simulink model "MATE_9LevelDrive_LowHarmonicRectifier"  (R2024b)
settings: Solver=FixedStepDiscrete  StartTime=0.0  StopTime=1  FixedStep=Ts  RelTol=1e-3
PostLoadFcn:
  | Ts=25e-6; initDrive9Level;Rsnu=30; Csnu=3e-6;Ron=0.01;Roff=1e6; Vf=2;
InitFcn:
  | Ts=25e-6; initDrive9Level;Rsnu=30; Csnu=3e-6;Ron=0.01;Roff=1e6; Vf=2;
values from neighbouring files (symbols this model uses):
  Lbase = Zbase/wbase    (= 0.0044902914611)    [initDrive9Level.m]
  Rgnd_rectifier = 1e4    (= 10000)    [initDrive9Level.m]
  T_2wind_ratio = 0.2677    [initDrive9Level.m]
  T_Lpu = Ltot_pu*9/10    (= 0.036)    [initDrive9Level.m]
  T_Lpu_pri = Ltot_pu/10    (= 0.004)    [initDrive9Level.m]
  T_Rpu = Rtot_pu*9/10    (= 0.009)    [initDrive9Level.m]
  T_Rpu_pri = Rtot_pu/10    (= 0.001)    [initDrive9Level.m]
  T_Vpri = 3000    [initDrive9Level.m]
  T_Vpri_15comp = 1.1168    [initDrive9Level.m]
  T_Vsec = 920    [initDrive9Level.m]
  Zbase = T_Vsec*T_Vsec/T_Pbase    (= 1.6928)    [initDrive9Level.m]
undefined symbols (not defined in the file or in its folder): DiscIntNeverNeededParam, gcbh, sps_rtmsupport
libraries: fl_lib x192, ee_lib x105, simetranss x26, nesl_utility x21
(part 3 of 5)

== system MATE_9LevelDrive_LowHarmonicRectifier/SSC multiwinding tranformer ==
  Electrical Reference : fl_lib/Electrical/Electrical Elements/Electrical Reference
  Electrical Reference1 : fl_lib/Electrical/Electrical Elements/Electrical Reference
  Electrical Reference2 : fl_lib/Electrical/Electrical Elements/Electrical Reference
  Phase Splitter{,4..7} (5 alike) : ee_lib/Connectors & References/Phase Splitter
  Seven-winding Decoupling Transformer : simetranss/Network decoupling/Seven-winding Decoupling Transformer  Tag=PublishSubsystem  Vpri=T_Vpri/sqrt(3)  RLpri=[T_Rpu_pri*Zbase T_Lpu_pri*Lbase]  Vwdn="[ T_Vsec/sqrt(3) T_Vsec T_Vsec/sqrt(3)*T_Vpri_15comp T_Vsec/sqrt(3)*T_2wind_ratio*T_Vpri_15comp T_Vsec/sqrt(3)*T_Vpri_15comp T_Vsec/sqrt(3)*T_2wind_ratio*T_Vpri_15comp  ]"  Lwdn="[T_Lpu_pri   T_Lpu T_Lpu T_Lpu*T_Vpri_15comp  T_Lpu*T_2wind_ratio*T_Vpri_15comp T_Lpu*T_Vpri_15comp  T_Lpu*T_2wind_ratio*T_Vpri_15comp ]*Lbase"  Rwdn="[     T_Rpu            T_Rpu    T_Rpu*T_Vpri_15comp T_Rpu*T_2wind_ratio*T_Vpri_15comp T_Rpu*T_Vpri_15comp T_Rpu*T_2wind_ratio*T_Vpri_15comp]*Zbase"  Rearth=1e6  Ts=Ts
  Seven-winding Decoupling Transformer1 : simetranss/Network decoupling/Seven-winding Decoupling Transformer  Tag=PublishSubsystem  Vpri=T_Vpri/sqrt(3)  RLpri=[T_Rpu_pri*Zbase T_Lpu_pri*Lbase]  Vwdn="[ T_Vsec/sqrt(3) T_Vsec T_Vsec/sqrt(3)*T_Vpri_15comp T_Vsec/sqrt(3)*T_2wind_ratio*T_Vpri_15comp T_Vsec/sqrt(3)*T_Vpri_15comp T_Vsec/sqrt(3)*T_2wind_ratio*T_Vpri_15comp  ]"  Lwdn="[T_Lpu_pri   T_Lpu T_Lpu T_Lpu*T_Vpri_15comp  T_Lpu*T_2wind_ratio*T_Vpri_15comp T_Lpu*T_Vpri_15comp  T_Lpu*T_2wind_ratio*T_Vpri_15comp ]*Lbase"  Rwdn="[     T_Rpu            T_Rpu    T_Rpu*T_Vpri_15comp T_Rpu*T_2wind_ratio*T_Vpri_15comp T_Rpu*T_Vpri_15comp T_Rpu*T_2wind_ratio*T_Vpri_15comp]*Zbase"  Rearth=1e6  Ts=Ts
  Seven-winding Decoupling Transformer2 : simetranss/Network decoupling/Seven-winding Decoupling Transformer  Tag=PublishSubsystem  Vpri=T_Vpri/sqrt(3)  RLpri=[T_Rpu_pri*Zbase T_Lpu_pri*Lbase]  Vwdn="[ T_Vsec/sqrt(3) T_Vsec T_Vsec/sqrt(3)*T_Vpri_15comp T_Vsec/sqrt(3)*T_2wind_ratio*T_Vpri_15comp T_Vsec/sqrt(3)*T_Vpri_15comp T_Vsec/sqrt(3)*T_2wind_ratio*T_Vpri_15comp  ]"  Lwdn="[T_Lpu_pri   T_Lpu T_Lpu T_Lpu*T_Vpri_15comp  T_Lpu*T_2wind_ratio*T_Vpri_15comp T_Lpu*T_Vpri_15comp  T_Lpu*T_2wind_ratio*T_Vpri_15comp ]*Lbase"  Rwdn="[     T_Rpu            T_Rpu    T_Rpu*T_Vpri_15comp T_Rpu*T_2wind_ratio*T_Vpri_15comp T_Rpu*T_Vpri_15comp T_Rpu*T_2wind_ratio*T_Vpri_15comp]*Zbase"  Rearth=1e6  Ts=Ts
  abc : PMIOPort  Side=Left
  abc2 : PMIOPort  Port=2  Side=Right
  abc3 : PMIOPort  Port=3  Side=Right
  abc4 : PMIOPort  Port=4  Side=Right
  abc5 : PMIOPort  Port=5  Side=Right
  connections:
  Seven-winding Decoupling Transformer/LConn2 -- Electrical Reference/LConn1
  Seven-winding Decoupling Transformer1/LConn2 -- Electrical Reference1/LConn1
  Seven-winding Decoupling Transformer2/LConn2 -- Electrical Reference2/LConn1
  Seven-winding Decoupling Transformer1/RConn8 -- Seven-winding Decoupling Transformer/RConn8 -- Seven-winding Decoupling Transformer2/RConn8
  Phase Splitter6/RConn2 -- Seven-winding Decoupling Transformer1/RConn5
  Phase Splitter6/RConn3 -- Seven-winding Decoupling Transformer2/RConn5
  Phase Splitter5/RConn2 -- Seven-winding Decoupling Transformer1/RConn1
  Phase Splitter5/RConn3 -- Seven-winding Decoupling Transformer2/RConn1
  Phase Splitter5/RConn1 -- Seven-winding Decoupling Transformer/RConn1
  Seven-winding Decoupling Transformer1/RConn2 -- Seven-winding Decoupling Transformer/RConn2 -- Seven-winding Decoupling Transformer2/RConn2
  Seven-winding Decoupling Transformer2/RConn6 -- Seven-winding Decoupling Transformer/RConn7
  Seven-winding Decoupling Transformer2/RConn3 -- Seven-winding Decoupling Transformer1/RConn4 -- Phase Splitter4/RConn3
  Seven-winding Decoupling Transformer1/RConn12 -- Seven-winding Decoupling Transformer/RConn12 -- Seven-winding Decoupling Transformer2/RConn12
  Phase Splitter7/RConn1 -- Seven-winding Decoupling Transformer/RConn9
  Phase Splitter7/RConn2 -- Seven-winding Decoupling Transformer1/RConn9
  Phase Splitter7/RConn3 -- Seven-winding Decoupling Transformer2/RConn9
  Seven-winding Decoupling Transformer2/RConn10 -- Seven-winding Decoupling Transformer1/RConn11
  Seven-winding Decoupling Transformer1/RConn10 -- Seven-winding Decoupling Transformer/RConn11
  Seven-winding Decoupling Transformer2/RConn11 -- Seven-winding Decoupling Transformer/RConn10
  Seven-winding Decoupling Transformer1/RConn3 -- Seven-winding Decoupling Transformer/RConn4 -- Phase Splitter4/RConn2
  Seven-winding Decoupling Transformer2/RConn4 -- Seven-winding Decoupling Transformer/RConn3 -- Phase Splitter4/RConn1
  Seven-winding Decoupling Transformer1/RConn7 -- Seven-winding Decoupling Transformer/RConn6
  Phase Splitter6/RConn1 -- Seven-winding Decoupling Transformer/RConn5
  Seven-winding Decoupling Transformer2/RConn7 -- Seven-winding Decoupling Transformer1/RConn6
  Phase Splitter/RConn1 -- Seven-winding Decoupling Transformer/LConn1
  Seven-winding Decoupling Transformer1/LConn1 -- Phase Splitter/RConn2
  Phase Splitter/RConn3 -- Seven-winding Decoupling Transformer2/LConn1
  abc2/RConn1 -- Phase Splitter5/LConn1
  abc3/RConn1 -- Phase Splitter4/LConn1
  abc4/RConn1 -- Phase Splitter6/LConn1
  abc5/RConn1 -- Phase Splitter7/LConn1
  abc/RConn1 -- Phase Splitter/LConn1

== system MATE_9LevelDrive_LowHarmonicRectifier/SSC multiwinding tranformer1 ==
  Electrical Reference : fl_lib/Electrical/Electrical Elements/Electrical Reference
  Electrical Reference1 : fl_lib/Electrical/Electrical Elements/Electrical Reference
  Electrical Reference2 : fl_lib/Electrical/Electrical Elements/Electrical Reference
  Phase Splitter{,4..7} (5 alike) : ee_lib/Connectors & References/Phase Splitter
  Seven-winding Decoupling Transformer : simetranss/Network decoupling/Seven-winding Decoupling Transformer  Tag=PublishSubsystem  Vpri=T_Vpri/sqrt(3)  RLpri=[T_Rpu_pri*Zbase T_Lpu_pri*Lbase]  Vwdn="[ T_Vsec/sqrt(3) T_Vsec T_Vsec/sqrt(3)*T_Vpri_15comp T_Vsec/sqrt(3)*T_2wind_ratio*T_Vpri_15comp T_Vsec/sqrt(3)*T_Vpri_15comp T_Vsec/sqrt(3)*T_2wind_ratio*T_Vpri_15comp  ]"  Lwdn="[T_Lpu_pri   T_Lpu T_Lpu T_Lpu*T_Vpri_15comp  T_Lpu*T_2wind_ratio*T_Vpri_15comp T_Lpu*T_Vpri_15comp  T_Lpu*T_2wind_ratio*T_Vpri_15comp ]*Lbase"  Rwdn="[     T_Rpu            T_Rpu    T_Rpu*T_Vpri_15comp T_Rpu*T_2wind_ratio*T_Vpri_15comp T_Rpu*T_Vpri_15comp T_Rpu*T_2wind_ratio*T_Vpri_15comp]*Zbase"  Rearth=1e6  Ts=Ts
  Seven-winding Decoupling Transformer1 : simetranss/Network decoupling/Seven-winding Decoupling Transformer  Tag=PublishSubsystem  Vpri=T_Vpri/sqrt(3)  RLpri=[T_Rpu_pri*Zbase T_Lpu_pri*Lbase]  Vwdn="[ T_Vsec/sqrt(3) T_Vsec T_Vsec/sqrt(3)*T_Vpri_15comp T_Vsec/sqrt(3)*T_2wind_ratio*T_Vpri_15comp T_Vsec/sqrt(3)*T_Vpri_15comp T_Vsec/sqrt(3)*T_2wind_ratio*T_Vpri_15comp  ]"  Lwdn="[T_Lpu_pri   T_Lpu T_Lpu T_Lpu*T_Vpri_15comp  T_Lpu*T_2wind_ratio*T_Vpri_15comp T_Lpu*T_Vpri_15comp  T_Lpu*T_2wind_ratio*T_Vpri_15comp ]*Lbase"  Rwdn="[     T_Rpu            T_Rpu    T_Rpu*T_Vpri_15comp T_Rpu*T_2wind_ratio*T_Vpri_15comp T_Rpu*T_Vpri_15comp T_Rpu*T_2wind_ratio*T_Vpri_15comp]*Zbase"  Rearth=1e6  Ts=Ts
  Seven-winding Decoupling Transformer2 : simetranss/Network decoupling/Seven-winding Decoupling Transformer  Tag=PublishSubsystem  Vpri=T_Vpri/sqrt(3)  RLpri=[T_Rpu_pri*Zbase T_Lpu_pri*Lbase]  Vwdn="[ T_Vsec/sqrt(3) T_Vsec T_Vsec/sqrt(3)*T_Vpri_15comp T_Vsec/sqrt(3)*T_2wind_ratio*T_Vpri_15comp T_Vsec/sqrt(3)*T_Vpri_15comp T_Vsec/sqrt(3)*T_2wind_ratio*T_Vpri_15comp  ]"  Lwdn="[T_Lpu_pri   T_Lpu T_Lpu T_Lpu*T_Vpri_15comp  T_Lpu*T_2wind_ratio*T_Vpri_15comp T_Lpu*T_Vpri_15comp  T_Lpu*T_2wind_ratio*T_Vpri_15comp ]*Lbase"  Rwdn="[     T_Rpu            T_Rpu    T_Rpu*T_Vpri_15comp T_Rpu*T_2wind_ratio*T_Vpri_15comp T_Rpu*T_Vpri_15comp T_Rpu*T_2wind_ratio*T_Vpri_15comp]*Zbase"  Rearth=1e6  Ts=Ts
  abc : PMIOPort  Side=Left
  abc2 : PMIOPort  Port=2  Side=Right
  abc3 : PMIOPort  Port=3  Side=Right
  abc4 : PMIOPort  Port=4  Side=Right
  abc5 : PMIOPort  Port=5  Side=Right
  connections:
  abc5/RConn1 -- Phase Splitter7/LConn1
  abc4/RConn1 -- Phase Splitter6/LConn1
  abc3/RConn1 -- Phase Splitter4/LConn1
  abc2/RConn1 -- Phase Splitter5/LConn1
  Phase Splitter/RConn3 -- Seven-winding Decoupling Transformer2/LConn1
  Seven-winding Decoupling Transformer1/LConn1 -- Phase Splitter/RConn2
  Phase Splitter/RConn1 -- Seven-winding Decoupling Transformer/LConn1
  Seven-winding Decoupling Transformer2/RConn7 -- Seven-winding Decoupling Transformer1/RConn6
  Phase Splitter6/RConn1 -- Seven-winding Decoupling Transformer/RConn5
  Seven-winding Decoupling Transformer1/RConn7 -- Seven-winding Decoupling Transformer/RConn6
  Phase Splitter4/RConn1 -- Seven-winding Decoupling Transformer/RConn3 -- Seven-winding Decoupling Transformer2/RConn4
  Phase Splitter4/RConn2 -- Seven-winding Decoupling Transformer/RConn4 -- Seven-winding Decoupling Transformer1/RConn3
  Seven-winding Decoupling Transformer2/RConn11 -- Seven-winding Decoupling Transformer/RConn10
  Seven-winding Decoupling Transformer1/RConn10 -- Seven-winding Decoupling Transformer/RConn11
  Seven-winding Decoupling Transformer2/RConn10 -- Seven-winding Decoupling Transformer1/RConn11
  Phase Splitter7/RConn3 -- Seven-winding Decoupling Transformer2/RConn9
  Phase Splitter7/RConn2 -- Seven-winding Decoupling Transformer1/RConn9
  Phase Splitter7/RConn1 -- Seven-winding Decoupling Transformer/RConn9
  Seven-winding Decoupling Transformer2/RConn12 -- Seven-winding Decoupling Transformer/RConn12 -- Seven-winding Decoupling Transformer1/RConn12
  Phase Splitter4/RConn3 -- Seven-winding Decoupling Transformer1/RConn4 -- Seven-winding Decoupling Transformer2/RConn3
  Seven-winding Decoupling Transformer2/RConn6 -- Seven-winding Decoupling Transformer/RConn7
  Seven-winding Decoupling Transformer2/RConn2 -- Seven-winding Decoupling Transformer/RConn2 -- Seven-winding Decoupling Transformer1/RConn2
  Phase Splitter5/RConn1 -- Seven-winding Decoupling Transformer/RConn1
  Phase Splitter5/RConn3 -- Seven-winding Decoupling Transformer2/RConn1
  Phase Splitter5/RConn2 -- Seven-winding Decoupling Transformer1/RConn1
  Phase Splitter6/RConn3 -- Seven-winding Decoupling Transformer2/RConn5
  Phase Splitter6/RConn2 -- Seven-winding Decoupling Transformer1/RConn5
  Seven-winding Decoupling Transformer2/RConn8 -- Seven-winding Decoupling Transformer/RConn8 -- Seven-winding Decoupling Transformer1/RConn8
  Seven-winding Decoupling Transformer2/LConn2 -- Electrical Reference2/LConn1
  Seven-winding Decoupling Transformer1/LConn2 -- Electrical Reference1/LConn1
  Seven-winding Decoupling Transformer/LConn2 -- Electrical Reference/LConn1
  abc/RConn1 -- Phase Splitter/LConn1

== system MATE_9LevelDrive_LowHarmonicRectifier/SSC multiwinding tranformer2 ==
  Electrical Reference : fl_lib/Electrical/Electrical Elements/Electrical Reference
  Electrical Reference1 : fl_lib/Electrical/Electrical Elements/Electrical Reference
  Electrical Reference2 : fl_lib/Electrical/Electrical Elements/Electrical Reference
  Phase Splitter{,4..7} (5 alike) : ee_lib/Connectors & References/Phase Splitter
  Seven-winding Decoupling Transformer : simetranss/Network decoupling/Seven-winding Decoupling Transformer  Tag=PublishSubsystem  Vpri=T_Vpri/sqrt(3)  RLpri=[T_Rpu_pri*Zbase T_Lpu_pri*Lbase]  Vwdn="[ T_Vsec/sqrt(3) T_Vsec T_Vsec/sqrt(3)*T_Vpri_15comp T_Vsec/sqrt(3)*T_2wind_ratio*T_Vpri_15comp T_Vsec/sqrt(3)*T_Vpri_15comp T_Vsec/sqrt(3)*T_2wind_ratio*T_Vpri_15comp  ]"  Lwdn="[T_Lpu_pri   T_Lpu T_Lpu T_Lpu*T_Vpri_15comp  T_Lpu*T_2wind_ratio*T_Vpri_15comp T_Lpu*T_Vpri_15comp  T_Lpu*T_2wind_ratio*T_Vpri_15comp ]*Lbase"  Rwdn="[     T_Rpu            T_Rpu    T_Rpu*T_Vpri_15comp T_Rpu*T_2wind_ratio*T_Vpri_15comp T_Rpu*T_Vpri_15comp T_Rpu*T_2wind_ratio*T_Vpri_15comp]*Zbase"  Rearth=1e6  Ts=Ts
  Seven-winding Decoupling Transformer1 : simetranss/Network decoupling/Seven-winding Decoupling Transformer  Tag=PublishSubsystem  Vpri=T_Vpri/sqrt(3)  RLpri=[T_Rpu_pri*Zbase T_Lpu_pri*Lbase]  Vwdn="[ T_Vsec/sqrt(3) T_Vsec T_Vsec/sqrt(3)*T_Vpri_15comp T_Vsec/sqrt(3)*T_2wind_ratio*T_Vpri_15comp T_Vsec/sqrt(3)*T_Vpri_15comp T_Vsec/sqrt(3)*T_2wind_ratio*T_Vpri_15comp  ]"  Lwdn="[T_Lpu_pri   T_Lpu T_Lpu T_Lpu*T_Vpri_15comp  T_Lpu*T_2wind_ratio*T_Vpri_15comp T_Lpu*T_Vpri_15comp  T_Lpu*T_2wind_ratio*T_Vpri_15comp ]*Lbase"  Rwdn="[     T_Rpu            T_Rpu    T_Rpu*T_Vpri_15comp T_Rpu*T_2wind_ratio*T_Vpri_15comp T_Rpu*T_Vpri_15comp T_Rpu*T_2wind_ratio*T_Vpri_15comp]*Zbase"  Rearth=1e6  Ts=Ts
  Seven-winding Decoupling Transformer2 : simetranss/Network decoupling/Seven-winding Decoupling Transformer  Tag=PublishSubsystem  Vpri=T_Vpri/sqrt(3)  RLpri=[T_Rpu_pri*Zbase T_Lpu_pri*Lbase]  Vwdn="[ T_Vsec/sqrt(3) T_Vsec T_Vsec/sqrt(3)*T_Vpri_15comp T_Vsec/sqrt(3)*T_2wind_ratio*T_Vpri_15comp T_Vsec/sqrt(3)*T_Vpri_15comp T_Vsec/sqrt(3)*T_2wind_ratio*T_Vpri_15comp  ]"  Lwdn="[T_Lpu_pri   T_Lpu T_Lpu T_Lpu*T_Vpri_15comp  T_Lpu*T_2wind_ratio*T_Vpri_15comp T_Lpu*T_Vpri_15comp  T_Lpu*T_2wind_ratio*T_Vpri_15comp ]*Lbase"  Rwdn="[     T_Rpu            T_Rpu    T_Rpu*T_Vpri_15comp T_Rpu*T_2wind_ratio*T_Vpri_15comp T_Rpu*T_Vpri_15comp T_Rpu*T_2wind_ratio*T_Vpri_15comp]*Zbase"  Rearth=1e6  Ts=Ts
  abc : PMIOPort  Side=Left
  abc2 : PMIOPort  Port=2  Side=Right
  abc3 : PMIOPort  Port=3  Side=Right
  abc4 : PMIOPort  Port=4  Side=Right
  abc5 : PMIOPort  Port=5  Side=Right
  connections:
  Seven-winding Decoupling Transformer/LConn2 -- Electrical Reference/LConn1
  Seven-winding Decoupling Transformer1/LConn2 -- Electrical Reference1/LConn1
  Seven-winding Decoupling Transformer2/LConn2 -- Electrical Reference2/LConn1
  Seven-winding Decoupling Transformer1/RConn8 -- Seven-winding Decoupling Transformer/RConn8 -- Seven-winding Decoupling Transformer2/RConn8
  Phase Splitter6/RConn2 -- Seven-winding Decoupling Transformer1/RConn5
  Phase Splitter6/RConn3 -- Seven-winding Decoupling Transformer2/RConn5
  Phase Splitter5/RConn2 -- Seven-winding Decoupling Transformer1/RConn1
  Phase Splitter5/RConn3 -- Seven-winding Decoupling Transformer2/RConn1
  Phase Splitter5/RConn1 -- Seven-winding Decoupling Transformer/RConn1
  Seven-winding Decoupling Transformer1/RConn2 -- Seven-winding Decoupling Transformer/RConn2 -- Seven-winding Decoupling Transformer2/RConn2
  Seven-winding Decoupling Transformer2/RConn6 -- Seven-winding Decoupling Transformer/RConn7
  Seven-winding Decoupling Transformer2/RConn3 -- Seven-winding Decoupling Transformer1/RConn4 -- Phase Splitter4/RConn3
  Seven-winding Decoupling Transformer1/RConn12 -- Seven-winding Decoupling Transformer/RConn12 -- Seven-winding Decoupling Transformer2/RConn12
  Phase Splitter7/RConn1 -- Seven-winding Decoupling Transformer/RConn9
  Phase Splitter7/RConn2 -- Seven-winding Decoupling Transformer1/RConn9
  Phase Splitter7/RConn3 -- Seven-winding Decoupling Transformer2/RConn9
  Seven-winding Decoupling Transformer2/RConn10 -- Seven-winding Decoupling Transformer1/RConn11
  Seven-winding Decoupling Transformer1/RConn10 -- Seven-winding Decoupling Transformer/RConn11
  Seven-winding Decoupling Transformer2/RConn11 -- Seven-winding Decoupling Transformer/RConn10
  Seven-winding Decoupling Transformer1/RConn3 -- Seven-winding Decoupling Transformer/RConn4 -- Phase Splitter4/RConn2
  Seven-winding Decoupling Transformer2/RConn4 -- Seven-winding Decoupling Transformer/RConn3 -- Phase Splitter4/RConn1
  Seven-winding Decoupling Transformer1/RConn7 -- Seven-winding Decoupling Transformer/RConn6
  Phase Splitter6/RConn1 -- Seven-winding Decoupling Transformer/RConn5
  Seven-winding Decoupling Transformer2/RConn7 -- Seven-winding Decoupling Transformer1/RConn6
  Phase Splitter/RConn1 -- Seven-winding Decoupling Transformer/LConn1
  Seven-winding Decoupling Transformer1/LConn1 -- Phase Splitter/RConn2
  Phase Splitter/RConn3 -- Seven-winding Decoupling Transformer2/LConn1
  abc2/RConn1 -- Phase Splitter5/LConn1
  abc3/RConn1 -- Phase Splitter4/LConn1
  abc4/RConn1 -- Phase Splitter6/LConn1
  abc5/RConn1 -- Phase Splitter7/LConn1
  abc/RConn1 -- Phase Splitter/LConn1

== system MATE_9LevelDrive_LowHarmonicRectifier/Subsystem1 ==
  Electrical Reference1 : fl_lib/Electrical/Electrical Elements/Electrical Reference
  Resistor : fl_lib/Electrical/Electrical Elements/Resistor  R=Rr Ohm  i_specify=off  i_priority=None  i=0 A  i_nominal_specify=off  i_nominal_value=1  i_nominal_unit=A  v_specify=off  v_priority=None  v=0 V  v_nominal_specify=off  v_nominal_value=1  v_nominal_unit=V
  Conn1 : PMIOPort  Side=Right
  connections:
  Resistor/RConn1 -- Conn1/RConn1
  Electrical Reference1/LConn1 -- Resistor/LConn1

== system MATE_9LevelDrive_LowHarmonicRectifier/Subsystem10 ==
  Electrical Reference1 : fl_lib/Electrical/Electrical Elements/Electrical Reference
  Resistor : fl_lib/Electrical/Electrical Elements/Resistor  R=Rr Ohm  i_specify=off  i_priority=None  i=0 A  i_nominal_specify=off  i_nominal_value=1  i_nominal_unit=A  v_specify=off  v_priority=None  v=0 V  v_nominal_specify=off  v_nominal_value=1  v_nominal_unit=V
  Conn1 : PMIOPort  Side=Right
  connections:
  Resistor/RConn1 -- Conn1/RConn1
  Electrical Reference1/LConn1 -- Resistor/LConn1

== system MATE_9LevelDrive_LowHarmonicRectifier/Subsystem11 ==
  Electrical Reference1 : fl_lib/Electrical/Electrical Elements/Electrical Reference
  Resistor : fl_lib/Electrical/Electrical Elements/Resistor  R=Rr Ohm  i_specify=off  i_priority=None  i=0 A  i_nominal_specify=off  i_nominal_value=1  i_nominal_unit=A  v_specify=off  v_priority=None  v=0 V  v_nominal_specify=off  v_nominal_value=1  v_nominal_unit=V
  Conn1 : PMIOPort  Side=Right
  connections:
  Electrical Reference1/LConn1 -- Resistor/LConn1
  Resistor/RConn1 -- Conn1/RConn1

== system MATE_9LevelDrive_LowHarmonicRectifier/Subsystem12 ==
  Electrical Reference1 : fl_lib/Electrical/Electrical Elements/Electrical Reference
  Resistor : fl_lib/Electrical/Electrical Elements/Resistor  R=Rr Ohm  i_specify=off  i_priority=None  i=0 A  i_nominal_specify=off  i_nominal_value=1  i_nominal_unit=A  v_specify=off  v_priority=None  v=0 V  v_nominal_specify=off  v_nominal_value=1  v_nominal_unit=V
  Conn1 : PMIOPort  Side=Right
  connections:
  Resistor/RConn1 -- Conn1/RConn1
  Electrical Reference1/LConn1 -- Resistor/LConn1

== system MATE_9LevelDrive_LowHarmonicRectifier/Subsystem13 ==
  Electrical Reference1 : fl_lib/Electrical/Electrical Elements/Electrical Reference
  Resistor : fl_lib/Electrical/Electrical Elements/Resistor  R=Rr Ohm  i_specify=off  i_priority=None  i=0 A  i_nominal_specify=off  i_nominal_value=1  i_nominal_unit=A  v_specify=off  v_priority=None  v=0 V  v_nominal_specify=off  v_nominal_value=1  v_nominal_unit=V
  Conn1 : PMIOPort  Side=Right
  connections:
  Electrical Reference1/LConn1 -- Resistor/LConn1
  Resistor/RConn1 -- Conn1/RConn1

== system MATE_9LevelDrive_LowHarmonicRectifier/Subsystem14 ==
  Electrical Reference1 : fl_lib/Electrical/Electrical Elements/Electrical Reference
  Resistor : fl_lib/Electrical/Electrical Elements/Resistor  R=Rr Ohm  i_specify=off  i_priority=None  i=0 A  i_nominal_specify=off  i_nominal_value=1  i_nominal_unit=A  v_specify=off  v_priority=None  v=0 V  v_nominal_specify=off  v_nominal_value=1  v_nominal_unit=V
  Conn1 : PMIOPort  Side=Right
  connections:
  Resistor/RConn1 -- Conn1/RConn1
  Electrical Reference1/LConn1 -- Resistor/LConn1

== system MATE_9LevelDrive_LowHarmonicRectifier/Subsystem2 ==
  Electrical Reference1 : fl_lib/Electrical/Electrical Elements/Electrical Reference
  Resistor : fl_lib/Electrical/Electrical Elements/Resistor  R=Rr Ohm  i_specify=off  i_priority=None  i=0 A  i_nominal_specify=off  i_nominal_value=1  i_nominal_unit=A  v_specify=off  v_priority=None  v=0 V  v_nominal_specify=off  v_nominal_value=1  v_nominal_unit=V
  Conn1 : PMIOPort  Side=Right
  connections:
  Electrical Reference1/LConn1 -- Resistor/LConn1
  Resistor/RConn1 -- Conn1/RConn1

== system MATE_9LevelDrive_LowHarmonicRectifier/Subsystem3 ==
  Electrical Reference1 : fl_lib/Electrical/Electrical Elements/Electrical Reference
  Resistor : fl_lib/Electrical/Electrical Elements/Resistor  R=Rr Ohm  i_specify=off  i_priority=None  i=0 A  i_nominal_specify=off  i_nominal_value=1  i_nominal_unit=A  v_specify=off  v_priority=None  v=0 V  v_nominal_specify=off  v_nominal_value=1  v_nominal_unit=V
  Conn1 : PMIOPort  Side=Right
  connections:
  Electrical Reference1/LConn1 -- Resistor/LConn1
  Resistor/RConn1 -- Conn1/RConn1

== system MATE_9LevelDrive_LowHarmonicRectifier/Subsystem4 ==
  Electrical Reference1 : fl_lib/Electrical/Electrical Elements/Electrical Reference
  Resistor : fl_lib/Electrical/Electrical Elements/Resistor  R=Rr Ohm  i_specify=off  i_priority=None  i=0 A  i_nominal_specify=off  i_nominal_value=1  i_nominal_unit=A  v_specify=off  v_priority=None  v=0 V  v_nominal_specify=off  v_nominal_value=1  v_nominal_unit=V
  Conn1 : PMIOPort  Side=Right
  connections:
  Resistor/RConn1 -- Conn1/RConn1
  Electrical Reference1/LConn1 -- Resistor/LConn1

== system MATE_9LevelDrive_LowHarmonicRectifier/Subsystem6 ==
  Electrical Reference1 : fl_lib/Electrical/Electrical Elements/Electrical Reference
  Resistor : fl_lib/Electrical/Electrical Elements/Resistor  R=Rr Ohm  i_specify=off  i_priority=None  i=0 A  i_nominal_specify=off  i_nominal_value=1  i_nominal_unit=A  v_specify=off  v_priority=None  v=0 V  v_nominal_specify=off  v_nominal_value=1  v_nominal_unit=V
  Conn1 : PMIOPort  Side=Right
  connections:
  Resistor/RConn1 -- Conn1/RConn1
  Electrical Reference1/LConn1 -- Resistor/LConn1

== system MATE_9LevelDrive_LowHarmonicRectifier/Subsystem7 ==
  Electrical Reference1 : fl_lib/Electrical/Electrical Elements/Electrical Reference
  Resistor : fl_lib/Electrical/Electrical Elements/Resistor  R=Rr Ohm  i_specify=off  i_priority=None  i=0 A  i_nominal_specify=off  i_nominal_value=1  i_nominal_unit=A  v_specify=off  v_priority=None  v=0 V  v_nominal_specify=off  v_nominal_value=1  v_nominal_unit=V
  Conn1 : PMIOPort  Side=Right
  connections:
  Electrical Reference1/LConn1 -- Resistor/LConn1
  Resistor/RConn1 -- Conn1/RConn1

== system MATE_9LevelDrive_LowHarmonicRectifier/Subsystem8 ==
  Electrical Reference1 : fl_lib/Electrical/Electrical Elements/Electrical Reference
  Resistor : fl_lib/Electrical/Electrical Elements/Resistor  R=Rr Ohm  i_specify=off  i_priority=None  i=0 A  i_nominal_specify=off  i_nominal_value=1  i_nominal_unit=A  v_specify=off  v_priority=None  v=0 V  v_nominal_specify=off  v_nominal_value=1  v_nominal_unit=V
  Conn1 : PMIOPort  Side=Right
  connections:
  Resistor/RConn1 -- Conn1/RConn1
  Electrical Reference1/LConn1 -- Resistor/LConn1

== system MATE_9LevelDrive_LowHarmonicRectifier/Subsystem9 ==
  Electrical Reference1 : fl_lib/Electrical/Electrical Elements/Electrical Reference
  Resistor : fl_lib/Electrical/Electrical Elements/Resistor  R=Rr Ohm  i_specify=off  i_priority=None  i=0 A  i_nominal_specify=off  i_nominal_value=1  i_nominal_unit=A  v_specify=off  v_priority=None  v=0 V  v_nominal_specify=off  v_nominal_value=1  v_nominal_unit=V
  Conn1 : PMIOPort  Side=Right
  connections:
  Electrical Reference1/LConn1 -- Resistor/LConn1
  Resistor/RConn1 -- Conn1/RConn1

== system MATE_9LevelDrive_LowHarmonicRectifier/backEMF ==
  amp : Inport
  freq : Inport  Port=2
  Constant1 : Constant  Value=2*pi/3
  Discrete-Time Integrator : DiscreteIntegrator  SampleTime=Ts  ICPrevOutput=DiscIntNeverNeededParam  ICPrevScaledInput=DiscIntNeverNeededParam
  Gain3 : Gain  Gain=2*pi
  Mux6 : Mux  Inputs=3
  Product2 : Product  RndMeth=Zero
  Sum : Sum  Inputs=+-
  Sum1 : Sum
  Trigonometric Function : Trigonometry
  Trigonometric Function1 : Trigonometry
  Trigonometric Function2 : Trigonometry
  Out1 : Outport  VectorParamsAs1DForOutWhenUnconnected=off
  wires:
  amp/1 -> Product2/1
  Mux6/1 -> Product2/2
  Trigonometric Function/1 -> Mux6/1
  Sum1/1 -> Trigonometric Function2/1
  Constant1/1 -> Sum1/2, Sum/2
  Sum/1 -> Trigonometric Function1/1
  Gain3/1 -> Discrete-Time Integrator/1
  Discrete-Time Integrator/1 -> Sum1/1, Sum/1, Trigonometric Function/1
  Product2/1 -> Out1/1
  freq/1 -> Gain3/1
  Trigonometric Function2/1 -> Mux6/3
  Trigonometric Function1/1 -> Mux6/2

== system MATE_9LevelDrive_LowHarmonicRectifier/Diode Bridge with snubber1/RCsnuber ==
  Capacitor : fl_lib/Electrical/Electrical Elements/Capacitor  c=Csnu F  r=0 Ohm  g=0 1/Ohm  i_specify=off  i_priority=None  i=0 A  i_nominal_specify=off  i_nominal_value=1  i_nominal_unit=A  v_specify=off  v_priority=None  v=0 V  v_nominal_specify=off  v_nominal_value=1  v_nominal_unit=V  vc_specify=off  vc_priority=High  vc=0 V  vc_nominal_specify=off  vc_nominal_value=1  vc_nominal_unit=V
  Resistor : fl_lib/Electrical/Electrical Elements/Resistor  R=Rsnu Ohm  i_specify=off  i_priority=None  i=0 A  i_nominal_specify=off  i_nominal_value=1  i_nominal_unit=A  v_specify=off  v_priority=None  v=0 V  v_nominal_specify=off  v_nominal_value=1  v_nominal_unit=V
  + : PMIOPort  Side=Left
  - : PMIOPort  Port=2  Side=Right
  connections:
  Resistor/LConn1 -- Capacitor/RConn1
  Capacitor/LConn1 -- +/RConn1
  Resistor/RConn1 -- -/RConn1

== system MATE_9LevelDrive_LowHarmonicRectifier/Diode Bridge with snubber1/RCsnuber1 ==
  Capacitor : fl_lib/Electrical/Electrical Elements/Capacitor  c=Csnu F  r=0 Ohm  g=0 1/Ohm  i_specify=off  i_priority=None  i=0 A  i_nominal_specify=off  i_nominal_value=1  i_nominal_unit=A  v_specify=off  v_priority=None  v=0 V  v_nominal_specify=off  v_nominal_value=1  v_nominal_unit=V  vc_specify=off  vc_priority=High  vc=0 V  vc_nominal_specify=off  vc_nominal_value=1  vc_nominal_unit=V
  Resistor : fl_lib/Electrical/Electrical Elements/Resistor  R=Rsnu Ohm  i_specify=off  i_priority=None  i=0 A  i_nominal_specify=off  i_nominal_value=1  i_nominal_unit=A  v_specify=off  v_priority=None  v=0 V  v_nominal_specify=off  v_nominal_value=1  v_nominal_unit=V
  + : PMIOPort  Side=Left
  - : PMIOPort  Port=2  Side=Right
  connections:
  Resistor/RConn1 -- -/RConn1
  Capacitor/LConn1 -- +/RConn1
  Resistor/LConn1 -- Capacitor/RConn1

== system MATE_9LevelDrive_LowHarmonicRectifier/Diode Bridge with snubber1/RCsnuber2 ==
  Capacitor : fl_lib/Electrical/Electrical Elements/Capacitor  c=Csnu F  r=0 Ohm  g=0 1/Ohm  i_specify=off  i_priority=None  i=0 A  i_nominal_specify=off  i_nominal_value=1  i_nominal_unit=A  v_specify=off  v_priority=None  v=0 V  v_nominal_specify=off  v_nominal_value=1  v_nominal_unit=V  vc_specify=off  vc_priority=High  vc=0 V  vc_nominal_specify=off  vc_nominal_value=1  vc_nominal_unit=V
  Resistor : fl_lib/Electrical/Electrical Elements/Resistor  R=Rsnu Ohm  i_specify=off  i_priority=None  i=0 A  i_nominal_specify=off  i_nominal_value=1  i_nominal_unit=A  v_specify=off  v_priority=None  v=0 V  v_nominal_specify=off  v_nominal_value=1  v_nominal_unit=V
  + : PMIOPort  Side=Left
  - : PMIOPort  Port=2  Side=Right
  connections:
  Resistor/LConn1 -- Capacitor/RConn1
  Capacitor/LConn1 -- +/RConn1
  Resistor/RConn1 -- -/RConn1

== system MATE_9LevelDrive_LowHarmonicRectifier/Diode Bridge with snubber1/RCsnuber3 ==
  Capacitor : fl_lib/Electrical/Electrical Elements/Capacitor  c=Csnu F  r=0 Ohm  g=0 1/Ohm  i_specify=off  i_priority=None  i=0 A  i_nominal_specify=off  i_nominal_value=1  i_nominal_unit=A  v_specify=off  v_priority=None  v=0 V  v_nominal_specify=off  v_nominal_value=1  v_nominal_unit=V  vc_specify=off  vc_priority=High  vc=0 V  vc_nominal_specify=off  vc_nominal_value=1  vc_nominal_unit=V
  Resistor : fl_lib/Electrical/Electrical Elements/Resistor  R=Rsnu Ohm  i_specify=off  i_priority=None  i=0 A  i_nominal_specify=off  i_nominal_value=1  i_nominal_unit=A  v_specify=off  v_priority=None  v=0 V  v_nominal_specify=off  v_nominal_value=1  v_nominal_unit=V
  + : PMIOPort  Side=Left
  - : PMIOPort  Port=2  Side=Right
  connections:
  Resistor/RConn1 -- -/RConn1
  Capacitor/LConn1 -- +/RConn1
  Resistor/LConn1 -- Capacitor/RConn1

== system MATE_9LevelDrive_LowHarmonicRectifier/Diode Bridge with snubber1/RCsnuber4 ==
  Capacitor : fl_lib/Electrical/Electrical Elements/Capacitor  c=Csnu F  r=0 Ohm  g=0 1/Ohm  i_specify=off  i_priority=None  i=0 A  i_nominal_specify=off  i_nominal_value=1  i_nominal_unit=A  v_specify=off  v_priority=None  v=0 V  v_nominal_specify=off  v_nominal_value=1  v_nominal_unit=V  vc_specify=off  vc_priority=High  vc=0 V  vc_nominal_specify=off  vc_nominal_value=1  vc_nominal_unit=V
  Resistor : fl_lib/Electrical/Electrical Elements/Resistor  R=Rsnu Ohm  i_specify=off  i_priority=None  i=0 A  i_nominal_specify=off  i_nominal_value=1  i_nominal_unit=A  v_specify=off  v_priority=None  v=0 V  v_nominal_specify=off  v_nominal_value=1  v_nominal_unit=V
  + : PMIOPort  Side=Left
  - : PMIOPort  Port=2  Side=Right
  connections:
  Resistor/RConn1 -- -/RConn1
  Capacitor/LConn1 -- +/RConn1
  Resistor/LConn1 -- Capacitor/RConn1

== system MATE_9LevelDrive_LowHarmonicRectifier/Diode Bridge with snubber1/RCsnuber5 ==
  Capacitor : fl_lib/Electrical/Electrical Elements/Capacitor  c=Csnu F  r=0 Ohm  g=0 1/Ohm  i_specify=off  i_priority=None  i=0 A  i_nominal_specify=off  i_nominal_value=1  i_nominal_unit=A  v_specify=off  v_priority=None  v=0 V  v_nominal_specify=off  v_nominal_value=1  v_nominal_unit=V  vc_specify=off  vc_priority=High  vc=0 V  vc_nominal_specify=off  vc_nominal_value=1  vc_nominal_unit=V
  Resistor : fl_lib/Electrical/Electrical Elements/Resistor  R=Rsnu Ohm  i_specify=off  i_priority=None  i=0 A  i_nominal_specify=off  i_nominal_value=1  i_nominal_unit=A  v_specify=off  v_priority=None  v=0 V  v_nominal_specify=off  v_nominal_value=1  v_nominal_unit=V
  + : PMIOPort  Side=Left
  - : PMIOPort  Port=2  Side=Right
  connections:
  Resistor/LConn1 -- Capacitor/RConn1
  Capacitor/LConn1 -- +/RConn1
  Resistor/RConn1 -- -/RConn1

== system MATE_9LevelDrive_LowHarmonicRectifier/Diode Bridge with snubber10/RCsnuber ==
  Capacitor : fl_lib/Electrical/Electrical Elements/Capacitor  c=Csnu F  r=0 Ohm  g=0 1/Ohm  i_specify=off  i_priority=None  i=0 A  i_nominal_specify=off  i_nominal_value=1  i_nominal_unit=A  v_specify=off  v_priority=None  v=0 V  v_nominal_specify=off  v_nominal_value=1  v_nominal_unit=V  vc_specify=off  vc_priority=High  vc=0 V  vc_nominal_specify=off  vc_nominal_value=1  vc_nominal_unit=V
  Resistor : fl_lib/Electrical/Electrical Elements/Resistor  R=Rsnu Ohm  i_specify=off  i_priority=None  i=0 A  i_nominal_specify=off  i_nominal_value=1  i_nominal_unit=A  v_specify=off  v_priority=None  v=0 V  v_nominal_specify=off  v_nominal_value=1  v_nominal_unit=V
  + : PMIOPort  Side=Left
  - : PMIOPort  Port=2  Side=Right
  connections:
  Resistor/RConn1 -- -/RConn1
  Capacitor/LConn1 -- +/RConn1
  Resistor/LConn1 -- Capacitor/RConn1

== system MATE_9LevelDrive_LowHarmonicRectifier/Diode Bridge with snubber10/RCsnuber1 ==
  Capacitor : fl_lib/Electrical/Electrical Elements/Capacitor  c=Csnu F  r=0 Ohm  g=0 1/Ohm  i_specify=off  i_priority=None  i=0 A  i_nominal_specify=off  i_nominal_value=1  i_nominal_unit=A  v_specify=off  v_priority=None  v=0 V  v_nominal_specify=off  v_nominal_value=1  v_nominal_unit=V  vc_specify=off  vc_priority=High  vc=0 V  vc_nominal_specify=off  vc_nominal_value=1  vc_nominal_unit=V
  Resistor : fl_lib/Electrical/Electrical Elements/Resistor  R=Rsnu Ohm  i_specify=off  i_priority=None  i=0 A  i_nominal_specify=off  i_nominal_value=1  i_nominal_unit=A  v_specify=off  v_priority=None  v=0 V  v_nominal_specify=off  v_nominal_value=1  v_nominal_unit=V
  + : PMIOPort  Side=Left
  - : PMIOPort  Port=2  Side=Right
  connections:
  Resistor/LConn1 -- Capacitor/RConn1
  Capacitor/LConn1 -- +/RConn1
  Resistor/RConn1 -- -/RConn1

== system MATE_9LevelDrive_LowHarmonicRectifier/Diode Bridge with snubber10/RCsnuber2 ==
  Capacitor : fl_lib/Electrical/Electrical Elements/Capacitor  c=Csnu F  r=0 Ohm  g=0 1/Ohm  i_specify=off  i_priority=None  i=0 A  i_nominal_specify=off  i_nominal_value=1  i_nominal_unit=A  v_specify=off  v_priority=None  v=0 V  v_nominal_specify=off  v_nominal_value=1  v_nominal_unit=V  vc_specify=off  vc_priority=High  vc=0 V  vc_nominal_specify=off  vc_nominal_value=1  vc_nominal_unit=V
  Resistor : fl_lib/Electrical/Electrical Elements/Resistor  R=Rsnu Ohm  i_specify=off  i_priority=None  i=0 A  i_nominal_specify=off  i_nominal_value=1  i_nominal_unit=A  v_specify=off  v_priority=None  v=0 V  v_nominal_specify=off  v_nominal_value=1  v_nominal_unit=V
  + : PMIOPort  Side=Left
  - : PMIOPort  Port=2  Side=Right
  connections:
  Resistor/RConn1 -- -/RConn1
  Capacitor/LConn1 -- +/RConn1
  Resistor/LConn1 -- Capacitor/RConn1

== system MATE_9LevelDrive_LowHarmonicRectifier/Diode Bridge with snubber10/RCsnuber3 ==
  Capacitor : fl_lib/Electrical/Electrical Elements/Capacitor  c=Csnu F  r=0 Ohm  g=0 1/Ohm  i_specify=off  i_priority=None  i=0 A  i_nominal_specify=off  i_nominal_value=1  i_nominal_unit=A  v_specify=off  v_priority=None  v=0 V  v_nominal_specify=off  v_nominal_value=1  v_nominal_unit=V  vc_specify=off  vc_priority=High  vc=0 V  vc_nominal_specify=off  vc_nominal_value=1  vc_nominal_unit=V
  Resistor : fl_lib/Electrical/Electrical Elements/Resistor  R=Rsnu Ohm  i_specify=off  i_priority=None  i=0 A  i_nominal_specify=off  i_nominal_value=1  i_nominal_unit=A  v_specify=off  v_priority=None  v=0 V  v_nominal_specify=off  v_nominal_value=1  v_nominal_unit=V
  + : PMIOPort  Side=Left
  - : PMIOPort  Port=2  Side=Right
  connections:
  Resistor/LConn1 -- Capacitor/RConn1
  Capacitor/LConn1 -- +/RConn1
  Resistor/RConn1 -- -/RConn1

== system MATE_9LevelDrive_LowHarmonicRectifier/Diode Bridge with snubber10/RCsnuber4 ==
  Capacitor : fl_lib/Electrical/Electrical Elements/Capacitor  c=Csnu F  r=0 Ohm  g=0 1/Ohm  i_specify=off  i_priority=None  i=0 A  i_nominal_specify=off  i_nominal_value=1  i_nominal_unit=A  v_specify=off  v_priority=None  v=0 V  v_nominal_specify=off  v_nominal_value=1  v_nominal_unit=V  vc_specify=off  vc_priority=High  vc=0 V  vc_nominal_specify=off  vc_nominal_value=1  vc_nominal_unit=V
  Resistor : fl_lib/Electrical/Electrical Elements/Resistor  R=Rsnu Ohm  i_specify=off  i_priority=None  i=0 A  i_nominal_specify=off  i_nominal_value=1  i_nominal_unit=A  v_specify=off  v_priority=None  v=0 V  v_nominal_specify=off  v_nominal_value=1  v_nominal_unit=V
  + : PMIOPort  Side=Left
  - : PMIOPort  Port=2  Side=Right
  connections:
  Resistor/LConn1 -- Capacitor/RConn1
  Capacitor/LConn1 -- +/RConn1
  Resistor/RConn1 -- -/RConn1

== system MATE_9LevelDrive_LowHarmonicRectifier/Diode Bridge with snubber10/RCsnuber5 ==
  Capacitor : fl_lib/Electrical/Electrical Elements/Capacitor  c=Csnu F  r=0 Ohm  g=0 1/Ohm  i_specify=off  i_priority=None  i=0 A  i_nominal_specify=off  i_nominal_value=1  i_nominal_unit=A  v_specify=off  v_priority=None  v=0 V  v_nominal_specify=off  v_nominal_value=1  v_nominal_unit=V  vc_specify=off  vc_priority=High  vc=0 V  vc_nominal_specify=off  vc_nominal_value=1  vc_nominal_unit=V
  Resistor : fl_lib/Electrical/Electrical Elements/Resistor  R=Rsnu Ohm  i_specify=off  i_priority=None  i=0 A  i_nominal_specify=off  i_nominal_value=1  i_nominal_unit=A  v_specify=off  v_priority=None  v=0 V  v_nominal_specify=off  v_nominal_value=1  v_nominal_unit=V
  + : PMIOPort  Side=Left
  - : PMIOPort  Port=2  Side=Right
  connections:
  Resistor/RConn1 -- -/RConn1
  Capacitor/LConn1 -- +/RConn1
  Resistor/LConn1 -- Capacitor/RConn1

== system MATE_9LevelDrive_LowHarmonicRectifier/Diode Bridge with snubber11/RCsnuber ==
  Capacitor : fl_lib/Electrical/Electrical Elements/Capacitor  c=Csnu F  r=0 Ohm  g=0 1/Ohm  i_specify=off  i_priority=None  i=0 A  i_nominal_specify=off  i_nominal_value=1  i_nominal_unit=A  v_specify=off  v_priority=None  v=0 V  v_nominal_specify=off  v_nominal_value=1  v_nominal_unit=V  vc_specify=off  vc_priority=High  vc=0 V  vc_nominal_specify=off  vc_nominal_value=1  vc_nominal_unit=V
  Resistor : fl_lib/Electrical/Electrical Elements/Resistor  R=Rsnu Ohm  i_specify=off  i_priority=None  i=0 A  i_nominal_specify=off  i_nominal_value=1  i_nominal_unit=A  v_specify=off  v_priority=None  v=0 V  v_nominal_specify=off  v_nominal_value=1  v_nominal_unit=V
  + : PMIOPort  Side=Left
  - : PMIOPort  Port=2  Side=Right
  connections:
  Resistor/LConn1 -- Capacitor/RConn1
  Capacitor/LConn1 -- +/RConn1
  Resistor/RConn1 -- -/RConn1

== system MATE_9LevelDrive_LowHarmonicRectifier/Diode Bridge with snubber11/RCsnuber1 ==
  Capacitor : fl_lib/Electrical/Electrical Elements/Capacitor  c=Csnu F  r=0 Ohm  g=0 1/Ohm  i_specify=off  i_priority=None  i=0 A  i_nominal_specify=off  i_nominal_value=1  i_nominal_unit=A  v_specify=off  v_priority=None  v=0 V  v_nominal_specify=off  v_nominal_value=1  v_nominal_unit=V  vc_specify=off  vc_priority=High  vc=0 V  vc_nominal_specify=off  vc_nominal_value=1  vc_nominal_unit=V
  Resistor : fl_lib/Electrical/Electrical Elements/Resistor  R=Rsnu Ohm  i_specify=off  i_priority=None  i=0 A  i_nominal_specify=off  i_nominal_value=1  i_nominal_unit=A  v_specify=off  v_priority=None  v=0 V  v_nominal_specify=off  v_nominal_value=1  v_nominal_unit=V
  + : PMIOPort  Side=Left
  - : PMIOPort  Port=2  Side=Right
  connections:
  Resistor/RConn1 -- -/RConn1
  Capacitor/LConn1 -- +/RConn1
  Resistor/LConn1 -- Capacitor/RConn1

== system MATE_9LevelDrive_LowHarmonicRectifier/Diode Bridge with snubber11/RCsnuber2 ==
  Capacitor : fl_lib/Electrical/Electrical Elements/Capacitor  c=Csnu F  r=0 Ohm  g=0 1/Ohm  i_specify=off  i_priority=None  i=0 A  i_nominal_specify=off  i_nominal_value=1  i_nominal_unit=A  v_specify=off  v_priority=None  v=0 V  v_nominal_specify=off  v_nominal_value=1  v_nominal_unit=V  vc_specify=off  vc_priority=High  vc=0 V  vc_nominal_specify=off  vc_nominal_value=1  vc_nominal_unit=V
  Resistor : fl_lib/Electrical/Electrical Elements/Resistor  R=Rsnu Ohm  i_specify=off  i_priority=None  i=0 A  i_nominal_specify=off  i_nominal_value=1  i_nominal_unit=A  v_specify=off  v_priority=None  v=0 V  v_nominal_specify=off  v_nominal_value=1  v_nominal_unit=V
  + : PMIOPort  Side=Left
  - : PMIOPort  Port=2  Side=Right
  connections:
  Resistor/LConn1 -- Capacitor/RConn1
  Capacitor/LConn1 -- +/RConn1
  Resistor/RConn1 -- -/RConn1

== system MATE_9LevelDrive_LowHarmonicRectifier/Diode Bridge with snubber11/RCsnuber3 ==
  Capacitor : fl_lib/Electrical/Electrical Elements/Capacitor  c=Csnu F  r=0 Ohm  g=0 1/Ohm  i_specify=off  i_priority=None  i=0 A  i_nominal_specify=off  i_nominal_value=1  i_nominal_unit=A  v_specify=off  v_priority=None  v=0 V  v_nominal_specify=off  v_nominal_value=1  v_nominal_unit=V  vc_specify=off  vc_priority=High  vc=0 V  vc_nominal_specify=off  vc_nominal_value=1  vc_nominal_unit=V
  Resistor : fl_lib/Electrical/Electrical Elements/Resistor  R=Rsnu Ohm  i_specify=off  i_priority=None  i=0 A  i_nominal_specify=off  i_nominal_value=1  i_nominal_unit=A  v_specify=off  v_priority=None  v=0 V  v_nominal_specify=off  v_nominal_value=1  v_nominal_unit=V
  + : PMIOPort  Side=Left
  - : PMIOPort  Port=2  Side=Right
  connections:
  Resistor/RConn1 -- -/RConn1
  Capacitor/LConn1 -- +/RConn1
  Resistor/LConn1 -- Capacitor/RConn1

== system MATE_9LevelDrive_LowHarmonicRectifier/Diode Bridge with snubber11/RCsnuber4 ==
  Capacitor : fl_lib/Electrical/Electrical Elements/Capacitor  c=Csnu F  r=0 Ohm  g=0 1/Ohm  i_specify=off  i_priority=None  i=0 A  i_nominal_specify=off  i_nominal_value=1  i_nominal_unit=A  v_specify=off  v_priority=None  v=0 V  v_nominal_specify=off  v_nominal_value=1  v_nominal_unit=V  vc_specify=off  vc_priority=High  vc=0 V  vc_nominal_specify=off  vc_nominal_value=1  vc_nominal_unit=V
  Resistor : fl_lib/Electrical/Electrical Elements/Resistor  R=Rsnu Ohm  i_specify=off  i_priority=None  i=0 A  i_nominal_specify=off  i_nominal_value=1  i_nominal_unit=A  v_specify=off  v_priority=None  v=0 V  v_nominal_specify=off  v_nominal_value=1  v_nominal_unit=V
  + : PMIOPort  Side=Left
  - : PMIOPort  Port=2  Side=Right
  connections:
  Resistor/RConn1 -- -/RConn1
  Capacitor/LConn1 -- +/RConn1
  Resistor/LConn1 -- Capacitor/RConn1

== system MATE_9LevelDrive_LowHarmonicRectifier/Diode Bridge with snubber11/RCsnuber5 ==
  Capacitor : fl_lib/Electrical/Electrical Elements/Capacitor  c=Csnu F  r=0 Ohm  g=0 1/Ohm  i_specify=off  i_priority=None  i=0 A  i_nominal_specify=off  i_nominal_value=1  i_nominal_unit=A  v_specify=off  v_priority=None  v=0 V  v_nominal_specify=off  v_nominal_value=1  v_nominal_unit=V  vc_specify=off  vc_priority=High  vc=0 V  vc_nominal_specify=off  vc_nominal_value=1  vc_nominal_unit=V
  Resistor : fl_lib/Electrical/Electrical Elements/Resistor  R=Rsnu Ohm  i_specify=off  i_priority=None  i=0 A  i_nominal_specify=off  i_nominal_value=1  i_nominal_unit=A  v_specify=off  v_priority=None  v=0 V  v_nominal_specify=off  v_nominal_value=1  v_nominal_unit=V
  + : PMIOPort  Side=Left
  - : PMIOPort  Port=2  Side=Right
  connections:
  Resistor/LConn1 -- Capacitor/RConn1
  Capacitor/LConn1 -- +/RConn1
  Resistor/RConn1 -- -/RConn1

== system MATE_9LevelDrive_LowHarmonicRectifier/Diode Bridge with snubber12/RCsnuber ==
  Capacitor : fl_lib/Electrical/Electrical Elements/Capacitor  c=Csnu F  r=0 Ohm  g=0 1/Ohm  i_specify=off  i_priority=None  i=0 A  i_nominal_specify=off  i_nominal_value=1  i_nominal_unit=A  v_specify=off  v_priority=None  v=0 V  v_nominal_specify=off  v_nominal_value=1  v_nominal_unit=V  vc_specify=off  vc_priority=High  vc=0 V  vc_nominal_specify=off  vc_nominal_value=1  vc_nominal_unit=V
  Resistor : fl_lib/Electrical/Electrical Elements/Resistor  R=Rsnu Ohm  i_specify=off  i_priority=None  i=0 A  i_nominal_specify=off  i_nominal_value=1  i_nominal_unit=A  v_specify=off  v_priority=None  v=0 V  v_nominal_specify=off  v_nominal_value=1  v_nominal_unit=V
  + : PMIOPort  Side=Left
  - : PMIOPort  Port=2  Side=Right
  connections:
  Resistor/RConn1 -- -/RConn1
  Capacitor/LConn1 -- +/RConn1
  Resistor/LConn1 -- Capacitor/RConn1

== system MATE_9LevelDrive_LowHarmonicRectifier/Diode Bridge with snubber12/RCsnuber1 ==
  Capacitor : fl_lib/Electrical/Electrical Elements/Capacitor  c=Csnu F  r=0 Ohm  g=0 1/Ohm  i_specify=off  i_priority=None  i=0 A  i_nominal_specify=off  i_nominal_value=1  i_nominal_unit=A  v_specify=off  v_priority=None  v=0 V  v_nominal_specify=off  v_nominal_value=1  v_nominal_unit=V  vc_specify=off  vc_priority=High  vc=0 V  vc_nominal_specify=off  vc_nominal_value=1  vc_nominal_unit=V
  Resistor : fl_lib/Electrical/Electrical Elements/Resistor  R=Rsnu Ohm  i_specify=off  i_priority=None  i=0 A  i_nominal_specify=off  i_nominal_value=1  i_nominal_unit=A  v_specify=off  v_priority=None  v=0 V  v_nominal_specify=off  v_nominal_value=1  v_nominal_unit=V
  + : PMIOPort  Side=Left
  - : PMIOPort  Port=2  Side=Right
  connections:
  Resistor/LConn1 -- Capacitor/RConn1
  Capacitor/LConn1 -- +/RConn1
  Resistor/RConn1 -- -/RConn1

== system MATE_9LevelDrive_LowHarmonicRectifier/Diode Bridge with snubber12/RCsnuber2 ==
  Capacitor : fl_lib/Electrical/Electrical Elements/Capacitor  c=Csnu F  r=0 Ohm  g=0 1/Ohm  i_specify=off  i_priority=None  i=0 A  i_nominal_specify=off  i_nominal_value=1  i_nominal_unit=A  v_specify=off  v_priority=None  v=0 V  v_nominal_specify=off  v_nominal_value=1  v_nominal_unit=V  vc_specify=off  vc_priority=High  vc=0 V  vc_nominal_specify=off  vc_nominal_value=1  vc_nominal_unit=V
  Resistor : fl_lib/Electrical/Electrical Elements/Resistor  R=Rsnu Ohm  i_specify=off  i_priority=None  i=0 A  i_nominal_specify=off  i_nominal_value=1  i_nominal_unit=A  v_specify=off  v_priority=None  v=0 V  v_nominal_specify=off  v_nominal_value=1  v_nominal_unit=V
  + : PMIOPort  Side=Left
  - : PMIOPort  Port=2  Side=Right
  connections:
  Resistor/RConn1 -- -/RConn1
  Capacitor/LConn1 -- +/RConn1
  Resistor/LConn1 -- Capacitor/RConn1

== system MATE_9LevelDrive_LowHarmonicRectifier/Diode Bridge with snubber12/RCsnuber3 ==
  Capacitor : fl_lib/Electrical/Electrical Elements/Capacitor  c=Csnu F  r=0 Ohm  g=0 1/Ohm  i_specify=off  i_priority=None  i=0 A  i_nominal_specify=off  i_nominal_value=1  i_nominal_unit=A  v_specify=off  v_priority=None  v=0 V  v_nominal_specify=off  v_nominal_value=1  v_nominal_unit=V  vc_specify=off  vc_priority=High  vc=0 V  vc_nominal_specify=off  vc_nominal_value=1  vc_nominal_unit=V
  Resistor : fl_lib/Electrical/Electrical Elements/Resistor  R=Rsnu Ohm  i_specify=off  i_priority=None  i=0 A  i_nominal_specify=off  i_nominal_value=1  i_nominal_unit=A  v_specify=off  v_priority=None  v=0 V  v_nominal_specify=off  v_nominal_value=1  v_nominal_unit=V
  + : PMIOPort  Side=Left
  - : PMIOPort  Port=2  Side=Right
  connections:
  Resistor/LConn1 -- Capacitor/RConn1
  Capacitor/LConn1 -- +/RConn1
  Resistor/RConn1 -- -/RConn1

== system MATE_9LevelDrive_LowHarmonicRectifier/Diode Bridge with snubber12/RCsnuber4 ==
  Capacitor : fl_lib/Electrical/Electrical Elements/Capacitor  c=Csnu F  r=0 Ohm  g=0 1/Ohm  i_specify=off  i_priority=None  i=0 A  i_nominal_specify=off  i_nominal_value=1  i_nominal_unit=A  v_specify=off  v_priority=None  v=0 V  v_nominal_specify=off  v_nominal_value=1  v_nominal_unit=V  vc_specify=off  vc_priority=High  vc=0 V  vc_nominal_specify=off  vc_nominal_value=1  vc_nominal_unit=V
  Resistor : fl_lib/Electrical/Electrical Elements/Resistor  R=Rsnu Ohm  i_specify=off  i_priority=None  i=0 A  i_nominal_specify=off  i_nominal_value=1  i_nominal_unit=A  v_specify=off  v_priority=None  v=0 V  v_nominal_specify=off  v_nominal_value=1  v_nominal_unit=V
  + : PMIOPort  Side=Left
  - : PMIOPort  Port=2  Side=Right
  connections:
  Resistor/LConn1 -- Capacitor/RConn1
  Capacitor/LConn1 -- +/RConn1
  Resistor/RConn1 -- -/RConn1

== system MATE_9LevelDrive_LowHarmonicRectifier/Diode Bridge with snubber12/RCsnuber5 ==
  Capacitor : fl_lib/Electrical/Electrical Elements/Capacitor  c=Csnu F  r=0 Ohm  g=0 1/Ohm  i_specify=off  i_priority=None  i=0 A  i_nominal_specify=off  i_nominal_value=1  i_nominal_unit=A  v_specify=off  v_priority=None  v=0 V  v_nominal_specify=off  v_nominal_value=1  v_nominal_unit=V  vc_specify=off  vc_priority=High  vc=0 V  vc_nominal_specify=off  vc_nominal_value=1  vc_nominal_unit=V
  Resistor : fl_lib/Electrical/Electrical Elements/Resistor  R=Rsnu Ohm  i_specify=off  i_priority=None  i=0 A  i_nominal_specify=off  i_nominal_value=1  i_nominal_unit=A  v_specify=off  v_priority=None  v=0 V  v_nominal_specify=off  v_nominal_value=1  v_nominal_unit=V
  + : PMIOPort  Side=Left
  - : PMIOPort  Port=2  Side=Right
  connections:
  Resistor/RConn1 -- -/RConn1
  Capacitor/LConn1 -- +/RConn1
  Resistor/LConn1 -- Capacitor/RConn1

== system MATE_9LevelDrive_LowHarmonicRectifier/Diode Bridge with snubber2/RCsnuber ==
  Capacitor : fl_lib/Electrical/Electrical Elements/Capacitor  c=Csnu F  r=0 Ohm  g=0 1/Ohm  i_specify=off  i_priority=None  i=0 A  i_nominal_specify=off  i_nominal_value=1  i_nominal_unit=A  v_specify=off  v_priority=None  v=0 V  v_nominal_specify=off  v_nominal_value=1  v_nominal_unit=V  vc_specify=off  vc_priority=High  vc=0 V  vc_nominal_specify=off  vc_nominal_value=1  vc_nominal_unit=V
  Resistor : fl_lib/Electrical/Electrical Elements/Resistor  R=Rsnu Ohm  i_specify=off  i_priority=None  i=0 A  i_nominal_specify=off  i_nominal_value=1  i_nominal_unit=A  v_specify=off  v_priority=None  v=0 V  v_nominal_specify=off  v_nominal_value=1  v_nominal_unit=V
  + : PMIOPort  Side=Left
  - : PMIOPort  Port=2  Side=Right
  connections:
  Resistor/RConn1 -- -/RConn1
  Capacitor/LConn1 -- +/RConn1
  Resistor/LConn1 -- Capacitor/RConn1

== system MATE_9LevelDrive_LowHarmonicRectifier/Diode Bridge with snubber2/RCsnuber1 ==
  Capacitor : fl_lib/Electrical/Electrical Elements/Capacitor  c=Csnu F  r=0 Ohm  g=0 1/Ohm  i_specify=off  i_priority=None  i=0 A  i_nominal_specify=off  i_nominal_value=1  i_nominal_unit=A  v_specify=off  v_priority=None  v=0 V  v_nominal_specify=off  v_nominal_value=1  v_nominal_unit=V  vc_specify=off  vc_priority=High  vc=0 V  vc_nominal_specify=off  vc_nominal_value=1  vc_nominal_unit=V
  Resistor : fl_lib/Electrical/Electrical Elements/Resistor  R=Rsnu Ohm  i_specify=off  i_priority=None  i=0 A  i_nominal_specify=off  i_nominal_value=1  i_nominal_unit=A  v_specify=off  v_priority=None  v=0 V  v_nominal_specify=off  v_nominal_value=1  v_nominal_unit=V
  + : PMIOPort  Side=Left
  - : PMIOPort  Port=2  Side=Right
  connections:
  Resistor/LConn1 -- Capacitor/RConn1
  Capacitor/LConn1 -- +/RConn1
  Resistor/RConn1 -- -/RConn1
